simulink model "VOOR"  (R2024a)
settings: Solver=FixedStepAuto  StartTime=0.0  StopTime=100  FixedStep=1e-3  RelTol=1e-3  EnableMultiTasking=on
undefined symbols (not defined in the file): D10, D11, D12, D2, D4, D5, D7, D8, D9, PTA0, PTA2, PTB23, PTB9, PTC3, PTC4, PTD0, PTD2, PTD3
libraries: frdmk64flib x10
settings Model: ExtModeTrigDuration=5  Creator=peter  LastModifiedBy=peter
settings OptimizationCC: EnhancedBackFolding=on  PassReuseOutputArgsAs=Individual arguments  ZeroExternalMemoryAtStartup=off  ZeroInternalMemoryAtStartup=off  MaxStackSize=64  OptimizeBlockOrder=speed  DifferentSizesBufferReuse=on  OptimizationCustomize=off  EfficientTunableParamExpr=on
settings DebuggingCC: ParameterTunabilityLossMsg=error
settings HardwareCC: ProdBitPerPointer=32  ProdBitPerSizeT=32  ProdBitPerPtrDiffT=32  ProdLargestAtomicInteger=Long  ProdLargestAtomicFloat=Double  ProdWordSize=32  ProdHWDeviceType=ARM Compatible->ARM Cortex
settings SFSimCC: MATLABDynamicMemAlloc=off
settings RTWCC: Description=Embedded Coder  SystemTargetFile=ert.tlc  HardwareBoard=NXP FRDM-K64F  TLCOptions="-aInlineSetEventsForThisBaseRateFcn=TLC_FALSE -aSuppressMultiTaskScheduler=TLC_FALSE  -aRateBasedStepFcn=0"  TemplateMakefile=ert_default_tmf  Toolchain=GNU Tools for ARM Embedded Processors
settings CodeAppCC: ForceParamTrailComments=on  IgnoreCustomStorageClasses=off  OperatorAnnotations=on  SimulinkDataObjDesc=on  SFDataObjDesc=on  InsertBlockDesc=on
settings ERTTargetCC: ExtModeTransport=4  ExtModeMexFile=sendToCommService

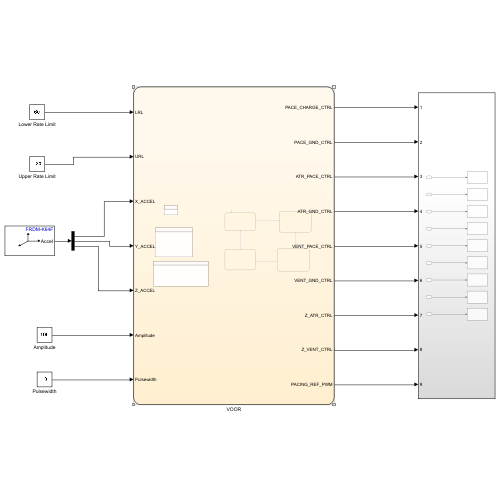
[thumbnail: Simulink's stored preview of the top-level diagram]
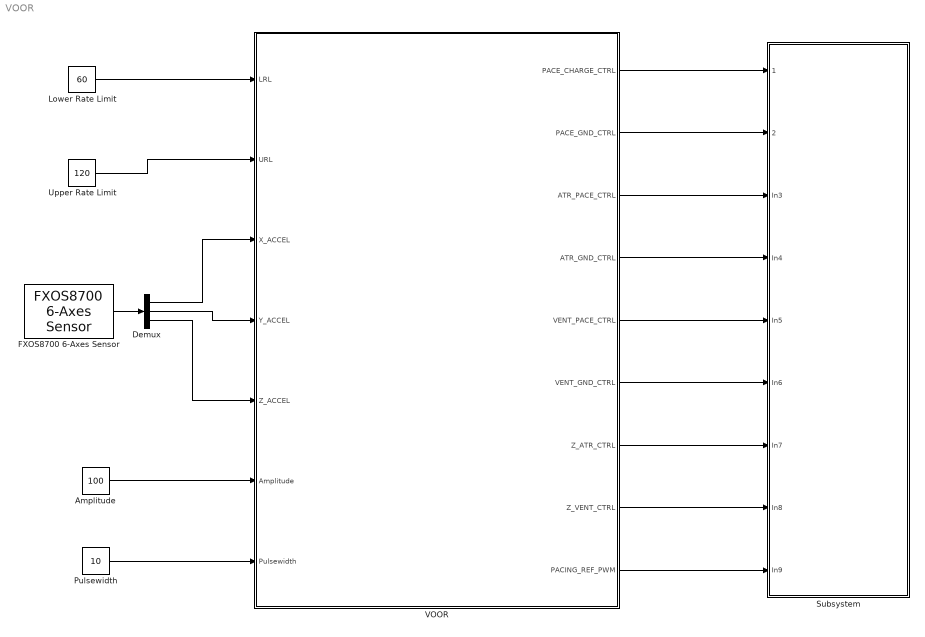
== system VOOR ==
  Amplitude : Constant  Value=100
  Demux : Demux  Outputs=3
  FXOS8700 6-Axes Sensor : frdmk64flib/FXOS8700 6-Axes Sensor  Activesensor=Accelerometer only  ODR=800Hz  HybridODR=400Hz  Accelfullrange=-4g to +4g  SampleTime=-1
  Lower Rate Limit : Constant  Value=60
  Pulsewidth : Constant  Value=10
  Subsystem : Subsystem
  Upper Rate Limit : Constant  Value=120
  VOOR : Stateflow chart  TreatAsAtomicUnit=on
  wires:
  Lower Rate Limit/1 -> VOOR/1(LRL)
  Amplitude/1 -> VOOR/6(Amplitude)
  Pulsewidth/1 -> VOOR/7(Pulsewidth)
  VOOR/1(PACE_CHARGE_CTRL) -> Subsystem/1(1)
  VOOR/2(PACE_GND_CTRL) -> Subsystem/2(2)
  VOOR/3(ATR_PACE_CTRL) -> Subsystem/3(In3)
  VOOR/4(ATR_GND_CTRL) -> Subsystem/4(In4)
  VOOR/5(VENT_PACE_CTRL) -> Subsystem/5(In5)
  VOOR/6(VENT_GND_CTRL) -> Subsystem/6(In6)
  VOOR/7(Z_ATR_CTRL) -> Subsystem/7(In7)
  VOOR/8(Z_VENT_CTRL) -> Subsystem/8(In8)
  VOOR/9(PACING_REF_PWM) -> Subsystem/9(In9)
  Upper Rate Limit/1 -> VOOR/2(URL)
  FXOS8700 6-Axes Sensor/1 -> Demux/1
  Demux/1 -> VOOR/3(X_ACCEL)
  Demux/3 -> VOOR/5(Z_ACCEL)
  Demux/2 -> VOOR/4(Y_ACCEL)

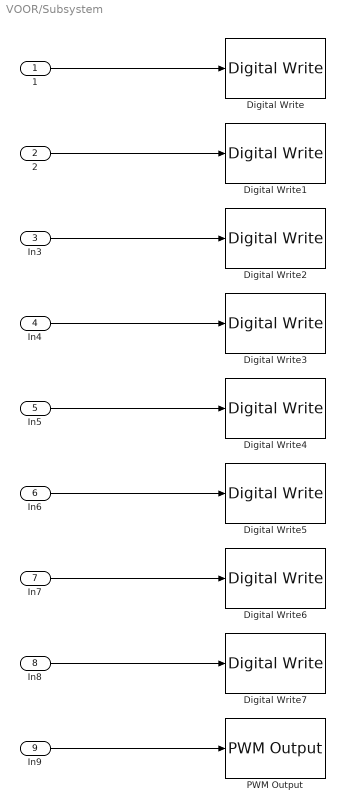
== system VOOR/Subsystem ==
  1 : Inport
  2 : Inport  Port=2
  In3 : Inport  Port=3
  In4 : Inport  Port=4
  In5 : Inport  Port=5
  In6 : Inport  Port=6
  In7 : Inport  Port=7
  In8 : Inport  Port=8
  In9 : Inport  Port=9
  Digital Write : frdmk64flib/Digital Write  Whichpin=PTB9 (D2)
  Digital Write1 : frdmk64flib/Digital Write  Whichpin=PTD0 (D10)
  Digital Write2 : frdmk64flib/Digital Write  Whichpin=PTA0 (D8)
  Digital Write3 : frdmk64flib/Digital Write  Whichpin=PTD2 (D11)
  Digital Write4 : frdmk64flib/Digital Write  Whichpin=PTC4 (D9)
  Digital Write5 : frdmk64flib/Digital Write  Whichpin=PTD3 (D12)
  Digital Write6 : frdmk64flib/Digital Write  Whichpin=PTB23 (D4)
  Digital Write7 : frdmk64flib/Digital Write  Whichpin=PTC3 (D7)
  PWM Output : frdmk64flib/PWM Output  Whichpin=PTA2 (D5)  InitialFrequency=2000  InitialDutyCycle=100
  wires:
  1/1 -> Digital Write/1
  2/1 -> Digital Write1/1
  In3/1 -> Digital Write2/1
  In4/1 -> Digital Write3/1
  In5/1 -> Digital Write4/1
  In6/1 -> Digital Write5/1
  In7/1 -> Digital Write6/1
  In8/1 -> Digital Write7/1
  In9/1 -> PWM Output/1

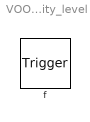
== system VOOR/VOOR/get_activity_level ==
  f : TriggerPort  TriggerType=function-call  VariantControl=(inherit)
      settings: CopyFcn=Stateflow.SLINSF.SimulinkMan.removeBlockPreDeleteFcn  PreDeleteFcn=Stateflow.SLINSF.SimulinkMan.unsafePredeleteFcn

== stateflow chart VOOR/VOOR ==
  state get_activity_level [function]
  state Pacing
    entry:
    PACE_CHARGE_CTRL=0;
    PACE_GND_CTRL=1;
    ATR_PACE_CTRL=0;
    ATR_GND_CTRL=0;
    Z_ATR_CTRL=0;
    Z_VENT_CTRL=0;
    VENT_GND_CTRL=0;
    VENT_PACE_CTRL=1;
  state Charging
    entry:
    ATR_PACE_CTRL=0;
    VENT_PACE_CTRL=0;
    PACING_REF_PWM=Amplitude;
    PACE_CHARGE_CTRL=1;
  state Discharging
    entry:
    PACE_GND_CTRL=1;
    VENT_PACE_CTRL=0;
    Z_ATR_CTRL=0;
    Z_VENT_CTRL=0;
    ATR_PACE_CTRL=0;
    ATR_GND_CTRL=0;
    VENT_GND_CTRL=1;
  state Calculate_new_rate
    entry:
    desired_rate = get_desired_rate();
    new_rate = get_controlled_rate();
  (default) -> Charging
  Charging -> Pacing : [after(60/LRL,sec)]
  Calculate_new_rate -> Charging
  Pacing -> Discharging : [after(Pulsewidth,msec)]
  Discharging -> Calculate_new_rate
  data: activity_level function_input; response_factor function_input; threshold function_input; desired_pace_rate function_input; current_rate function_input; reaction_time function_input; recovery_time function_input; LRL input; URL input; X_ACCEL input; Y_ACCEL input; Z_ACCEL input; Amplitude input; Pulsewidth input; PACE_CHARGE_CTRL output; PACE_GND_CTRL output; ATR_PACE_CTRL output; ATR_GND_CTRL output; VENT_PACE_CTRL output; VENT_GND_CTRL output; Z_ATR_CTRL output; Z_VENT_CTRL output; PACING_REF_PWM output
  function get_desired_rate(activity_level, response_factor, threshold):
    | function get_desired_rate(activity_level, response_factor, threshold)
    | 
    | xy = XY_ACCEL;
    | z = Z_ACCEL;
    | if xy > threshold
    |     
    | end 
    | 
    | if z > threshold
    |     
    | end 
    | 
    |     return desired_pacing_rate;
    | end
  function get_controlled_rate(desired_pace_rate,current_rate,reaction_time,recovery_time):
    | function get_controlled_rate(desired_pace_rate,current_rate,reaction_time,recovery_time)
    | 
    | 
    |     return new_rate
    | end
